simulink model "Sim_5"  (R2020b)
settings: Solver=VariableStepAuto  StartTime=0.0  StopTime=100000.0  RelTol=1e-3
values from neighbouring files (symbols this model uses):
  A_i = 56.5    [Projekt5.m]
  A_os = 56.5    [Projekt5.m]
  alfa_1 = 729.55    [Projekt5.m]
  alfa_2 = 6567.6    [Projekt5.m]
  beta_1 = -15000    [Projekt5.m]
  beta_2 = -20000    [Projekt5.m]
  c_m = 0.12    [Projekt5.m]
  c_p = 1    [Projekt5.m]
  h_i = 160/60    (= 2.66666666667)    [Projekt5.m]
  h_os = 1000/60    (= 16.6666666667)    [Projekt5.m]
  lambda_1 = -40000    [Projekt5.m]
  lambda_2 = -50000    [Projekt5.m]
  ro = 50    [Projekt5.m]
  ro_m = 512    [Projekt5.m]
  T_0 = 80    [Projekt5.m]
  T_m0 = 80    [Projekt5.m]
  Tj = 212    [Projekt5.m]
  V = 42.5    [Projekt5.m]
  V_m = 9.42    [Projekt5.m]
libraries: simulink x7
settings Model: Creator=Bartek  LastModifiedBy=Bartek

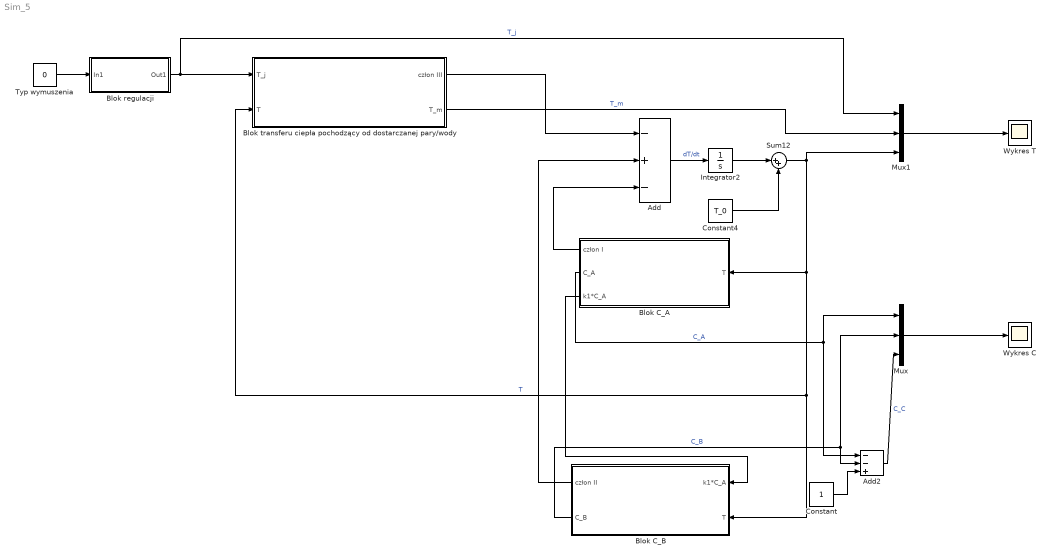
== system Sim_5 ==
  Add : Sum  Inputs=-+-
  Add2 : Sum  Inputs=--+
  Blok C_A : Subsystem
  Blok C_B : Subsystem
  Blok regulacji : Subsystem
  Blok transferu ciepła pochodzący od dostarczanej pary/wody : Subsystem
  Constant : Constant
  Constant4 : Constant  Value=T_0
  Integrator2 : Integrator
  Mux : Mux  Inputs=3
  Mux1 : Mux  Inputs=3
  Sum12 : Sum  Inputs=|++
  Typ wymuszenia : Constant  Value=0
  Wykres C : Scope
  Wykres T : Scope
  wires:
  Add/1 -> Integrator2/1  "dT/dt"
  Integrator2/1 -> Sum12/1
  Constant4/1 -> Sum12/2
  Sum12/1 -> Mux1/3, Blok C_B/2(T), Blok transferu ciepła pochodzący od dostarczanej pary/wody/2(T), Blok C_A/1(T)  "T"
  Mux/1 -> Wykres C/1
  Constant/1 -> Add2/3
  Add2/1 -> Mux/3  "C_C"
  Blok regulacji/1(Out1) -> Mux1/1, Blok transferu ciepła pochodzący od dostarczanej pary/wody/1(T_j)  "T_j"
  Mux1/1 -> Wykres T/1
  Typ wymuszenia/1 -> Blok regulacji/1(In1)
  Blok C_A/2(C_A) -> Mux/1, Add2/1  "C_A"
  Blok C_A/1(człon I) -> Add/3
  Blok C_B/2(C_B) -> Mux/2, Add2/2  "C_B"
  Blok C_A/3(k1*C_A) -> Blok C_B/1(k1*C_A)
  Blok C_B/1(człon II) -> Add/2
  Blok transferu ciepła pochodzący od dostarczanej pary/wody/1(człon III) -> Add/1
  Blok transferu ciepła pochodzący od dostarczanej pary/wody/2(T_m) -> Mux1/2  "T_m"

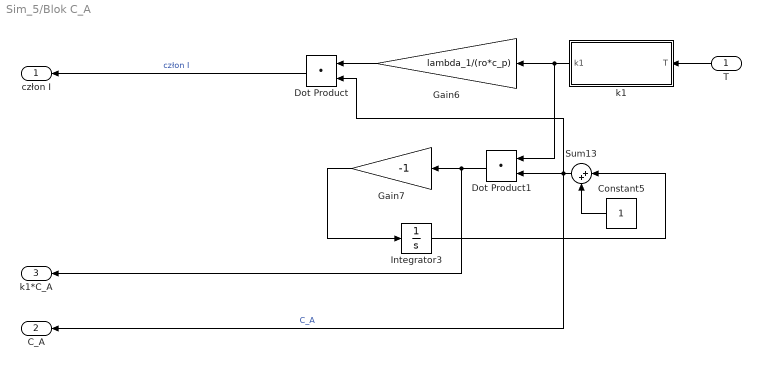
== system Sim_5/Blok C_A ==
  T : Inport
  Constant5 : Constant
  Dot Product : DotProduct  InputSameDT=on  OutDataTypeStr=Inherit: Inherit via internal rule
  Dot Product1 : DotProduct  InputSameDT=on  OutDataTypeStr=Inherit: Inherit via internal rule
  Gain6 : Gain  Gain=lambda_1/(ro*c_p)
  Gain7 : Gain  Gain=-1
  Integrator3 : Integrator
  Sum13 : Sum  Inputs=|++
  k1 : Subsystem
  człon I : Outport
  C_A : Outport  Port=2
  k1*C_A : Outport  Port=3
  wires:
  Dot Product/1 -> człon I/1  "człon I"
  Dot Product1/1 -> k1*C_A/1, Gain7/1
  k1/1(k1) -> Gain6/1, Dot Product1/1
  Gain7/1 -> Integrator3/1
  Sum13/1 -> Dot Product/2, C_A/1, Dot Product1/2  "C_A"
  Integrator3/1 -> Sum13/1
  Constant5/1 -> Sum13/2
  T/1 -> k1/1(T)
  Gain6/1 -> Dot Product/1

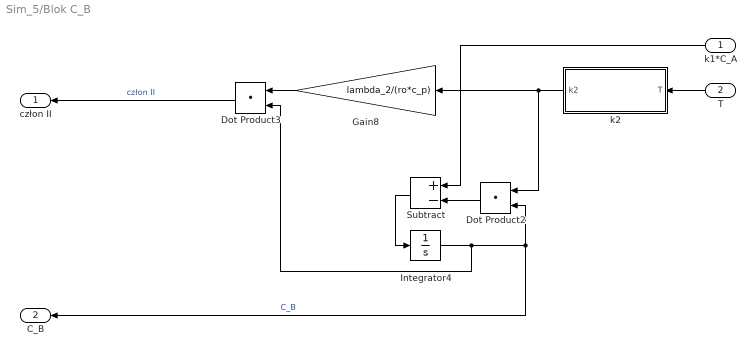
== system Sim_5/Blok C_B ==
  k1*C_A : Inport
  T : Inport  Port=2
  Dot Product2 : DotProduct  InputSameDT=on  OutDataTypeStr=Inherit: Inherit via internal rule
  Dot Product3 : DotProduct  InputSameDT=on  OutDataTypeStr=Inherit: Inherit via internal rule
  Gain8 : Gain  Gain=lambda_2/(ro*c_p)
  Integrator4 : Integrator
  Subtract : Sum  Inputs=+-
  k2 : Subsystem
  człon II : Outport
  C_B : Outport  Port=2
  wires:
  k2/1(k2) -> Gain8/1, Dot Product2/1
  Integrator4/1 -> C_B/1, Dot Product2/2, Dot Product3/2  "C_B"
  Gain8/1 -> Dot Product3/1
  Dot Product3/1 -> człon II/1  "człon II"
  T/1 -> k2/1(T)
  Dot Product2/1 -> Subtract/2
  k1*C_A/1 -> Subtract/1
  Subtract/1 -> Integrator4/1

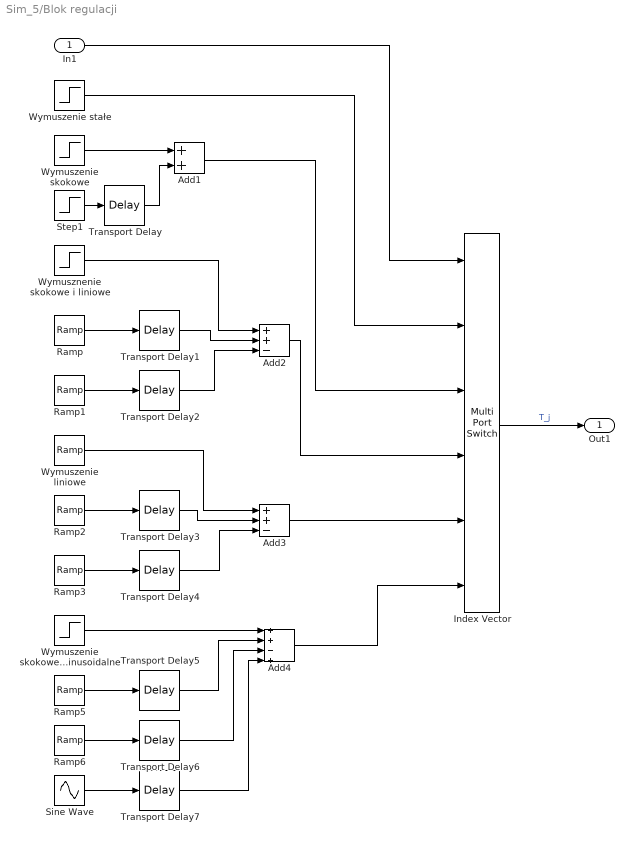
== system Sim_5/Blok regulacji ==
  In1 : Inport
  Add1 : Sum
  Add2 : Sum  Inputs=++-
  Add3 : Sum  Inputs=++-
  Add4 : Sum  Inputs=++-+
  Index Vector : MultiPortSwitch  DataPortOrder=Zero-based contiguous  Inputs=5  zeroidx=on
  Ramp{,1,3,5..6} (5 alike) : simulink/Sources/Ramp  slope=-2  start=0  InitialOutput=0
  Ramp2 : simulink/Sources/Ramp  slope=-7  start=0  InitialOutput=0
  Sine Wave : Sin  Amplitude=10  Frequency=0.01  SampleTime=0
  Step1 : Step  Time=0  After=-132  SampleTime=0
  Transport Delay : TransportDelay  DelayTime=40
  Transport Delay1 : TransportDelay  DelayTime=20
  Transport Delay2 : TransportDelay  DelayTime=100
  Transport Delay3 : TransportDelay  DelayTime=30
  Transport Delay4 : TransportDelay  DelayTime=80
  Transport Delay5 : TransportDelay  DelayTime=20
  Transport Delay6 : TransportDelay  DelayTime=80
  Transport Delay7 : TransportDelay  DelayTime=100
  Wymuszenie liniowe : simulink/Sources/Ramp  slope=5  start=0  InitialOutput=80
  Wymuszenie skokowe : Step  Time=0  After=Tj  SampleTime=0
  "Wymuszenie skokowe, liniowe i sinusoidalne" : Step  Time=0  After=Tj  SampleTime=0
  Wymuszenie stałe : Step  Time=0  After=0  SampleTime=0
  Wymusznenie skokowe i liniowe : Step  Time=0  After=Tj  SampleTime=0
  Out1 : Outport
  wires:
  In1/1 -> Index Vector/1
  Index Vector/1 -> Out1/1  "T_j"
  Add1/1 -> Index Vector/3
  Transport Delay/1 -> Add1/2
  Wymuszenie skokowe/1 -> Add1/1
  Step1/1 -> Transport Delay/1
  Wymuszenie stałe/1 -> Index Vector/2
  Wymusznenie skokowe i liniowe/1 -> Add2/1
  Ramp/1 -> Transport Delay1/1
  Transport Delay1/1 -> Add2/2
  Add2/1 -> Index Vector/4
  Ramp1/1 -> Transport Delay2/1
  Transport Delay2/1 -> Add2/3
  Transport Delay4/1 -> Add3/3
  Ramp2/1 -> Transport Delay3/1
  Ramp3/1 -> Transport Delay4/1
  Transport Delay3/1 -> Add3/2
  Wymuszenie liniowe/1 -> Add3/1
  Add3/1 -> Index Vector/5
  Transport Delay6/1 -> Add4/3
  "Wymuszenie skokowe, liniowe i sinusoidalne"/1 -> Add4/1
  Ramp5/1 -> Transport Delay5/1
  Ramp6/1 -> Transport Delay6/1
  Transport Delay5/1 -> Add4/2
  Add4/1 -> Index Vector/6
  Sine Wave/1 -> Transport Delay7/1
  Transport Delay7/1 -> Add4/4

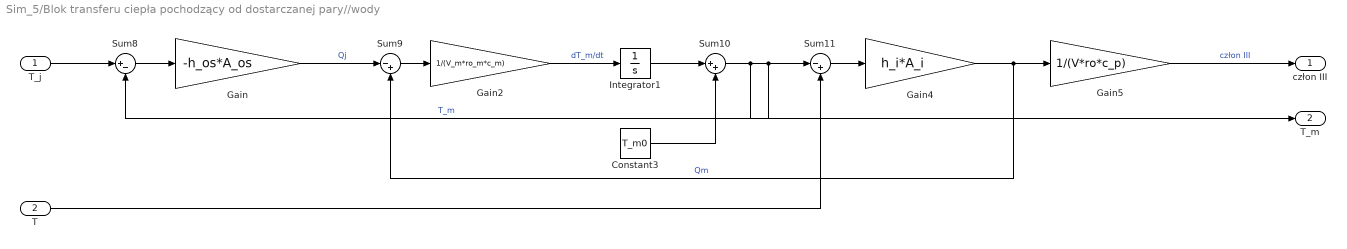
== system Sim_5/Blok transferu ciepła pochodzący od dostarczanej pary//wody ==
  T_j : Inport
  T : Inport  Port=2
  Constant3 : Constant  Value=T_m0
  Gain : Gain  Gain=-h_os*A_os
  Gain2 : Gain  Gain=1/(V_m*ro_m*c_m)
  Gain4 : Gain  Gain=h_i*A_i
  Gain5 : Gain  Gain=1/(V*ro*c_p)
  Integrator1 : Integrator
  Sum10 : Sum  Inputs=|++
  Sum11 : Sum  Inputs=|-+
  Sum8 : Sum  Inputs=|+-
  Sum9 : Sum  Inputs=|-+
  człon III : Outport
  T_m : Outport  Port=2
  wires:
  Integrator1/1 -> Sum10/1
  T_j/1 -> Sum8/1
  Sum10/1 -> T_m/1, Sum11/1, Sum8/2  "T_m"
  Sum9/1 -> Gain2/1
  Gain4/1 -> Sum9/2, Gain5/1  "Qm"
  Gain/1 -> Sum9/1  "Qj"
  Sum11/1 -> Gain4/1
  Gain2/1 -> Integrator1/1  "dT_m/dt"
  Constant3/1 -> Sum10/2
  Sum8/1 -> Gain/1
  Gain5/1 -> człon III/1  "człon III"
  T/1 -> Sum11/2

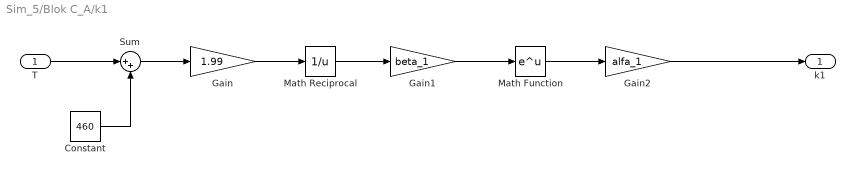
== system Sim_5/Blok C_A/k1 ==
  T : Inport
  Constant : Constant  Value=460
  Gain : Gain  Gain=1.99
  Gain1 : Gain  Gain=beta_1
  Gain2 : Gain  Gain=alfa_1
  Math Function : Math  SaturateOnIntegerOverflow=on
  Math Reciprocal : Math  Operator=reciprocal  SignedPower=on  SaturateOnIntegerOverflow=on
  Sum : Sum  Inputs=|++
  k1 : Outport
  wires:
  T/1 -> Sum/1
  Constant/1 -> Sum/2
  Sum/1 -> Gain/1
  Gain/1 -> Math Reciprocal/1
  Math Reciprocal/1 -> Gain1/1
  Gain1/1 -> Math Function/1
  Math Function/1 -> Gain2/1
  Gain2/1 -> k1/1

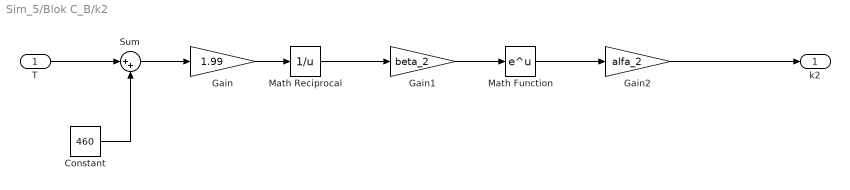
== system Sim_5/Blok C_B/k2 ==
  T : Inport
  Constant : Constant  Value=460
  Gain : Gain  Gain=1.99
  Gain1 : Gain  Gain=beta_2
  Gain2 : Gain  Gain=alfa_2
  Math Function : Math  SaturateOnIntegerOverflow=on
  Math Reciprocal : Math  Operator=reciprocal  SignedPower=on  SaturateOnIntegerOverflow=on
  Sum : Sum  Inputs=|++
  k2 : Outport
  wires:
  T/1 -> Sum/1
  Constant/1 -> Sum/2
  Sum/1 -> Gain/1
  Gain/1 -> Math Reciprocal/1
  Math Reciprocal/1 -> Gain1/1
  Gain1/1 -> Math Function/1
  Math Function/1 -> Gain2/1
  Gain2/1 -> k2/1
